simulink model "test"  (R2023b)
settings: Solver=VariableStepAuto  StartTime=0.0  StopTime=10.0  RelTol=1e-3
libraries: mcbcontrolslib x3, dspfdesign x3, slpidlib x3, spsSawtoothGeneratorLib x1, simulink x1, spsSVPWMGenerator2LevelLib x1
settings Model: Creator=LZQ  LastModifiedBy=LZQ

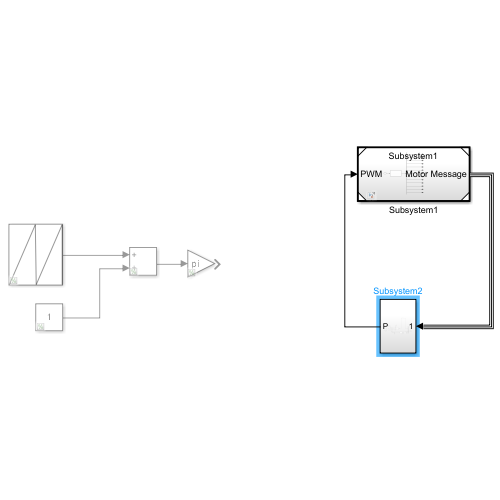
[thumbnail: Simulink's stored preview of the top-level diagram]
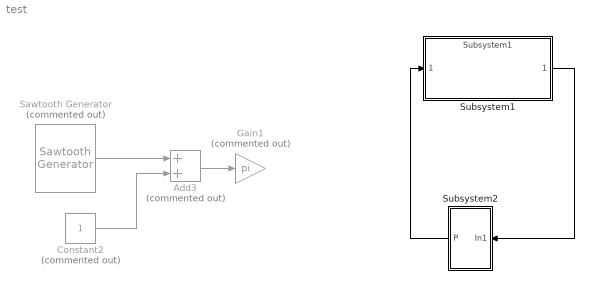
== system test ==
  Add3 : Sum  Commented=on
  Constant2 : Constant  Commented=on
  Gain1 : Gain  Commented=on  Gain=pi
  Sawtooth Generator : spsSawtoothGeneratorLib/Sawtooth Generator  Commented=on  Freq=1  Phase=360  Ts=0
  Subsystem1 : ModelReference  ModelNameDialog=Subsystem1  SimulationMode=Normal  ModelReferenceVersion=1.2
  Subsystem2 : Subsystem
  wires:
  Constant2/1 -> Add3/2
  Add3/1 -> Gain1/1
  Sawtooth Generator/1 -> Add3/1
  Subsystem1/1 -> Subsystem2/1(In1)
  Subsystem2/1(P) -> Subsystem1/1

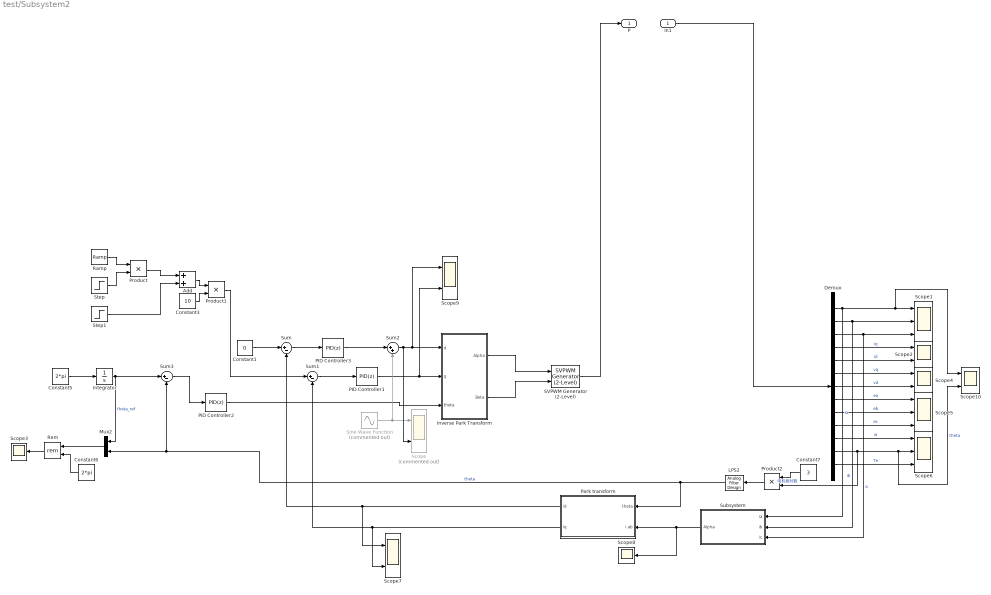
== system test/Subsystem2 ==
  In1 : Inport
  Add : Sum
  Constant1 : Constant  Value=0
  Constant3 : Constant  Value=10
  Constant5 : Constant  Value=2*pi
  Constant6 : Constant  Value=2*pi
  Constant7 : Constant  Value=3
  Demux : Demux  Outputs=13
  Integrator : Integrator
  Inverse Park Transform : Subsystem
  LPS2 : dspfdesign/Analog Filter Design  method=Butterworth  filttype=Lowpass  N=8  Wlo=30  Whi=80  Rp=2  Rs=40
  Mux2 : Mux  Inputs=2
  PID Controller1 : slpidlib/PID Controller  Controller=PID  Form=Parallel  TimeDomain=Discrete-time  UseExternalTs=off  SampleTime=1e-5  IntegratorMethod=Forward Euler  FilterMethod=Forward Euler  ControllerParametersSource=internal  P=0.000004  I=0.000001  UseKiTs=off  D=0  N=100  UseFilter=on  TunerSelectOption=Transfer Function Based (PID Tuner App)  InitialConditionSource=internal  InitialConditionForIntegrator=0  InitialConditionForFilter=0  DifferentiatorICPrevScaledInput=0  ExternalReset=none  TrackingMode=off  Kt=1  LimitOutput=off  SatLimitsSource=internal  UpperSaturationLimit=inf  LowerSaturationLimit=-inf  LinearizeAsGain=on  AntiWindupMode=none  Kb=1  LimitIntegrator=off  UpperIntegratorSaturationLimit=inf  LowerIntegratorSaturationLimit=-inf  POutMin=[]  POutMax=[]  IOutMin=[-0.001]  IOutMax=[0.001]  DOutMin=[]  DOutMax=[]  NOutMin=[]  NOutMax=[]  SumOutMin=[-0.01]  SumOutMax=[0.01]  SaturationOutMin=[]  SaturationOutMax=[]  PParamMin=[]  PParamMax=[]  IParamMin=[]  IParamMax=[]  DParamMin=[]  DParamMax=[]  NParamMin=[]  NParamMax=[]  KbParamMin=[]  KbParamMax=[]  KtParamMin=[]  KtParamMax=[]  KbOutMin=[]  KbOutMax=[]  KtOutMin=[]  KtOutMax=[]  IntegratorOutMin=[]  IntegratorOutMax=[]  FilterOutMin=[]  FilterOutMax=[]  SumI1OutMin=[]  SumI1OutMax=[]  SumI2OutMin=[]  SumI2OutMax=[]  SumI3OutMin=[]  SumI3OutMax=[]  SumI4OutMin=[]  SumI4OutMax=[]  SumDOutMin=[]  SumDOutMax=[]  DifferentiatorOutMin=[]  DifferentiatorOutMax=[]  FilterDiffOutCoefMin=[]  FilterDiffOutCoefMax=[]  ReciprocalOutMin=[]  ReciprocalOutMax=[]  SumDenOutMin=[]  SumDenOutMax=[]  SumNumOutMin=[]  SumNumOutMax=[]  DivideOutMin=[]  DivideOutMax=[]  UdiffTsProdOutMin=[]  UdiffTsProdOutMax=[]  NTsProdOutMin=[]  NTsProdOutMax=[]  UintegralTsProdOutMin=[]  UintegralTsProdOutMax=[]  UngainTsProdOutMin=[]  UngainTsProdOutMax=[]  ClampingZeroOutDataTypeStr=Inherit: Inherit via back propagation  ClampingZeroOutMin=[]  ClampingZeroOutMax=[]  FilterDenConstantOutDataTypeStr=Inherit: Inherit via back propagation  FilterDenConstantOutMin=[]  FilterDenConstantOutMax=[]  PCopyOutDataTypeStr=Inherit: Inherit via back propagation  PCopyOutMin=[]  PCopyOutMax=[]  NCopyOutDataTypeStr=Inherit: Inherit via back propagation  NCopyOutMin=[]  NCopyOutMax=[]  IntegratorContinuousStateAttributes=''  IntegratorStateMustResolveToSignalObject=off  IntegratorRTWStateStorageClass=Auto  FilterContinuousStateAttributes=''  FilterStateMustResolveToSignalObject=off  FilterRTWStateStorageClass=Auto  ParallelPVariant=InternalParameters  IdealPVariant=Disabled  IVariant=InternalParameters  DVariant=InternalParameters  IntegratorVariant=Discrete  SatVariant=Disabled  AWVariant=Passthrough  PCopyVariant=Disabled  TRVariant=Disabled  FdbkBlocksVariant=Forward  IdealPFdbkVariant=Disabled  SatFdbkVariant=Disabled  DerivativeFilterVariant=ForwardEulerFilter  NVariant=InternalParameters  NCopyVariant=Disabled  FilterICVariant=InternalICsFilter  IntegratorICVariant=InternalICs  ExternalResetVariant=Disabled  TRSumVariant=Passthrough  SumFdbkVariant=Disabled  SumVariant=Sum_PID  TsampFilterVariant=InternalTs  TsampNgainVariant=Passthrough  TsampIntegralVariant=Disabled_SignalSpec  ExternalSaturationOutDataTypeStr=Inherit: Same as second input
  PID Controller2 : slpidlib/PID Controller  Controller=PID  Form=Parallel  TimeDomain=Discrete-time  UseExternalTs=off  SampleTime=0.0005  IntegratorMethod=Forward Euler  FilterMethod=Forward Euler  ControllerParametersSource=internal  P=0.1  I=0.04  UseKiTs=off  D=0  N=100  UseFilter=on  TunerSelectOption=Transfer Function Based (PID Tuner App)  InitialConditionSource=internal  InitialConditionForIntegrator=0  InitialConditionForFilter=0  DifferentiatorICPrevScaledInput=0  ExternalReset=none  TrackingMode=off  Kt=1  LimitOutput=off  SatLimitsSource=internal  UpperSaturationLimit=inf  LowerSaturationLimit=-inf  LinearizeAsGain=on  AntiWindupMode=none  Kb=1  LimitIntegrator=off  UpperIntegratorSaturationLimit=inf  LowerIntegratorSaturationLimit=-inf  POutMin=[]  POutMax=[]  IOutMin=[]  IOutMax=[]  DOutMin=[]  DOutMax=[]  NOutMin=[]  NOutMax=[]  SumOutMin=[]  SumOutMax=[]  SaturationOutMin=[]  SaturationOutMax=[]  PParamMin=[]  PParamMax=[]  IParamMin=[]  IParamMax=[]  DParamMin=[]  DParamMax=[]  NParamMin=[]  NParamMax=[]  KbParamMin=[]  KbParamMax=[]  KtParamMin=[]  KtParamMax=[]  KbOutMin=[]  KbOutMax=[]  KtOutMin=[]  KtOutMax=[]  IntegratorOutMin=[]  IntegratorOutMax=[]  FilterOutMin=[]  FilterOutMax=[]  SumI1OutMin=[]  SumI1OutMax=[]  SumI2OutMin=[]  SumI2OutMax=[]  SumI3OutMin=[]  SumI3OutMax=[]  SumI4OutMin=[]  SumI4OutMax=[]  SumDOutMin=[]  SumDOutMax=[]  DifferentiatorOutMin=[]  DifferentiatorOutMax=[]  FilterDiffOutCoefMin=[]  FilterDiffOutCoefMax=[]  ReciprocalOutMin=[]  ReciprocalOutMax=[]  SumDenOutMin=[]  SumDenOutMax=[]  SumNumOutMin=[]  SumNumOutMax=[]  DivideOutMin=[]  DivideOutMax=[]  UdiffTsProdOutMin=[]  UdiffTsProdOutMax=[]  NTsProdOutMin=[]  NTsProdOutMax=[]  UintegralTsProdOutMin=[]  UintegralTsProdOutMax=[]  UngainTsProdOutMin=[]  UngainTsProdOutMax=[]  ClampingZeroOutDataTypeStr=Inherit: Inherit via back propagation  ClampingZeroOutMin=[]  ClampingZeroOutMax=[]  FilterDenConstantOutDataTypeStr=Inherit: Inherit via back propagation  FilterDenConstantOutMin=[]  FilterDenConstantOutMax=[]  PCopyOutDataTypeStr=Inherit: Inherit via back propagation  PCopyOutMin=[]  PCopyOutMax=[]  NCopyOutDataTypeStr=Inherit: Inherit via back propagation  NCopyOutMin=[]  NCopyOutMax=[]  IntegratorContinuousStateAttributes=''  IntegratorStateMustResolveToSignalObject=off  IntegratorRTWStateStorageClass=Auto  FilterContinuousStateAttributes=''  FilterStateMustResolveToSignalObject=off  FilterRTWStateStorageClass=Auto  ParallelPVariant=InternalParameters  IdealPVariant=Disabled  IVariant=InternalParameters  DVariant=InternalParameters  IntegratorVariant=Discrete  SatVariant=Disabled  AWVariant=Passthrough  PCopyVariant=Disabled  TRVariant=Disabled  FdbkBlocksVariant=Forward  IdealPFdbkVariant=Disabled  SatFdbkVariant=Disabled  DerivativeFilterVariant=ForwardEulerFilter  NVariant=InternalParameters  NCopyVariant=Disabled  FilterICVariant=InternalICsFilter  IntegratorICVariant=InternalICs  ExternalResetVariant=Disabled  TRSumVariant=Passthrough  SumFdbkVariant=Disabled  SumVariant=Sum_PID  TsampFilterVariant=InternalTs  TsampNgainVariant=Passthrough  TsampIntegralVariant=Disabled_SignalSpec  ExternalSaturationOutDataTypeStr=Inherit: Same as second input
  PID Controller3 : slpidlib/PID Controller  Controller=PID  Form=Parallel  TimeDomain=Discrete-time  UseExternalTs=off  SampleTime=1e-5  IntegratorMethod=Forward Euler  FilterMethod=Forward Euler  ControllerParametersSource=internal  P=0.000004  I=0.000001  UseKiTs=off  D=0  N=100  UseFilter=on  TunerSelectOption=Transfer Function Based (PID Tuner App)  InitialConditionSource=internal  InitialConditionForIntegrator=0  InitialConditionForFilter=0  DifferentiatorICPrevScaledInput=0  ExternalReset=none  TrackingMode=off  Kt=1  LimitOutput=off  SatLimitsSource=internal  UpperSaturationLimit=inf  LowerSaturationLimit=-inf  LinearizeAsGain=on  AntiWindupMode=none  Kb=1  LimitIntegrator=off  UpperIntegratorSaturationLimit=inf  LowerIntegratorSaturationLimit=-inf  POutMin=[]  POutMax=[]  IOutMin=[-0.001]  IOutMax=[0.001]  DOutMin=[]  DOutMax=[]  NOutMin=[]  NOutMax=[]  SumOutMin=[-0.01]  SumOutMax=[0.01]  SaturationOutMin=[]  SaturationOutMax=[]  PParamMin=[]  PParamMax=[]  IParamMin=[]  IParamMax=[]  DParamMin=[]  DParamMax=[]  NParamMin=[]  NParamMax=[]  KbParamMin=[]  KbParamMax=[]  KtParamMin=[]  KtParamMax=[]  KbOutMin=[]  KbOutMax=[]  KtOutMin=[]  KtOutMax=[]  IntegratorOutMin=[]  IntegratorOutMax=[]  FilterOutMin=[]  FilterOutMax=[]  SumI1OutMin=[]  SumI1OutMax=[]  SumI2OutMin=[]  SumI2OutMax=[]  SumI3OutMin=[]  SumI3OutMax=[]  SumI4OutMin=[]  SumI4OutMax=[]  SumDOutMin=[]  SumDOutMax=[]  DifferentiatorOutMin=[]  DifferentiatorOutMax=[]  FilterDiffOutCoefMin=[]  FilterDiffOutCoefMax=[]  ReciprocalOutMin=[]  ReciprocalOutMax=[]  SumDenOutMin=[]  SumDenOutMax=[]  SumNumOutMin=[]  SumNumOutMax=[]  DivideOutMin=[]  DivideOutMax=[]  UdiffTsProdOutMin=[]  UdiffTsProdOutMax=[]  NTsProdOutMin=[]  NTsProdOutMax=[]  UintegralTsProdOutMin=[]  UintegralTsProdOutMax=[]  UngainTsProdOutMin=[]  UngainTsProdOutMax=[]  ClampingZeroOutDataTypeStr=Inherit: Inherit via back propagation  ClampingZeroOutMin=[]  ClampingZeroOutMax=[]  FilterDenConstantOutDataTypeStr=Inherit: Inherit via back propagation  FilterDenConstantOutMin=[]  FilterDenConstantOutMax=[]  PCopyOutDataTypeStr=Inherit: Inherit via back propagation  PCopyOutMin=[]  PCopyOutMax=[]  NCopyOutDataTypeStr=Inherit: Inherit via back propagation  NCopyOutMin=[]  NCopyOutMax=[]  IntegratorContinuousStateAttributes=''  IntegratorStateMustResolveToSignalObject=off  IntegratorRTWStateStorageClass=Auto  FilterContinuousStateAttributes=''  FilterStateMustResolveToSignalObject=off  FilterRTWStateStorageClass=Auto  ParallelPVariant=InternalParameters  IdealPVariant=Disabled  IVariant=InternalParameters  DVariant=InternalParameters  IntegratorVariant=Discrete  SatVariant=Disabled  AWVariant=Passthrough  PCopyVariant=Disabled  TRVariant=Disabled  FdbkBlocksVariant=Forward  IdealPFdbkVariant=Disabled  SatFdbkVariant=Disabled  DerivativeFilterVariant=ForwardEulerFilter  NVariant=InternalParameters  NCopyVariant=Disabled  FilterICVariant=InternalICsFilter  IntegratorICVariant=InternalICs  ExternalResetVariant=Disabled  TRSumVariant=Passthrough  SumFdbkVariant=Disabled  SumVariant=Sum_PID  TsampFilterVariant=InternalTs  TsampNgainVariant=Passthrough  TsampIntegralVariant=Disabled_SignalSpec  ExternalSaturationOutDataTypeStr=Inherit: Same as second input
  Park transform : Subsystem
  Product : Product
  Product1 : Product
  Product2 : Product
  Ramp : simulink/Sources/Ramp  slope=0.2  start=0  InitialOutput=0.2
  Rem : Math  Operator=rem
  SVPWM Generator (2-Level) : spsSVPWMGenerator2LevelLib/SVPWM Generator (2-Level)  InputType=alpha-beta components  SwitchingPattern=Pattern #1  Fc=20000  ParUref=[0.8 -30 50]  Ts=0
  Scope : Scope  Commented=on  NumInputPorts=2
  Scope1 : Scope  NumInputPorts=3
  Scope{2,4,7,9..10} (5 alike) : Scope  NumInputPorts=2
  Scope3 : Scope
  Scope5 : Scope  NumInputPorts=3
  Scope6 : Scope  NumInputPorts=3
  Scope8 : Scope
  Sine Wave Function : Sin  Commented=on  Amplitude=0.2  Frequency=2*pi*800  Phase=pi/2  SampleTime=0.000005
  Step : Step  Time=4  Before=1  After=0  SampleTime=0
  Step1 : Step  Time=4  SampleTime=0
  Subsystem : Subsystem
  Sum : Sum  Inputs=|+-
  Sum1 : Sum  Inputs=|+-
  Sum2 : Sum  Inputs=|++
  Sum3 : Sum  Inputs=|+-
  P : Outport
  wires:
  PID Controller2/1 -> Inverse Park Transform/3(theta)
  Demux/1 -> Subsystem/1(ia), Scope10/1, Scope1/1  "ia"
  PID Controller1/1 -> Scope9/2, Inverse Park Transform/2(q)
  LPS2/1 -> Sum3/2, Mux2/2, Park transform/1(theta)  "theta"
  Inverse Park Transform/1(Alpha) -> SVPWM Generator (2-Level)/1
  Sine Wave Function/1 -> Sum2/2, Scope/1
  Demux/9 -> Scope5/2  "eb"
  Rem/1 -> Scope3/1
  Constant3/1 -> Product1/2
  Sum2/1 -> Scope9/1, Inverse Park Transform/1(d), Scope/2
  Demux/7 -> Scope4/2  "vd"
  Inverse Park Transform/2(Beta) -> SVPWM Generator (2-Level)/2
  Constant1/1 -> Sum/1
  Product/1 -> Add/1
  PID Controller3/1 -> Sum2/1
  Park transform/2(iq) -> Sum1/2, Scope7/2
  Sum1/1 -> PID Controller1/1
  Sum3/1 -> PID Controller2/1
  Constant7/1 -> Product2/1  "电机极对数"
  Park transform/1(id) -> Sum/2, Scope7/1
  Demux/12 -> Product2/2, Scope10/2, Scope6/2  "theta"
  Constant5/1 -> Integrator/1
  Add/1 -> Product1/1
  Demux/3 -> Subsystem/3(ic), Scope1/3  "ic"
  Integrator/1 -> Mux2/1, Sum3/1  "theta_ref"
  Demux/4 -> Scope2/1  "iq"
  Demux/2 -> Subsystem/2(ib), Scope1/2  "ib"
  Step1/1 -> Add/2
  Demux/13 -> Scope6/3  "Te"
  Subsystem/1(Alpha) -> Park transform/2(i ab), Scope8/1
  Ramp/1 -> Product/1
  Demux/10 -> Scope5/3  "ec"
  Mux2/1 -> Rem/1
  Constant6/1 -> Rem/2
  Demux/11 -> Scope6/1  "w"
  Demux/6 -> Scope4/1  "vq"
  Demux/5 -> Scope2/2  "id"
  Demux/8 -> Scope5/1  "ea"
  Product1/1 -> Sum1/1
  Sum/1 -> PID Controller3/1
  Step/1 -> Product/2
  Product2/1 -> LPS2/1
  SVPWM Generator (2-Level)/1 -> P/1
  In1/1 -> Demux/1

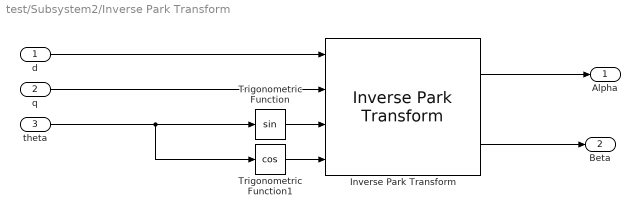
== system test/Subsystem2/Inverse Park Transform ==
  d : Inport  SampleTime=1e-5
  q : Inport  Port=2  SampleTime=1e-5
  theta : Inport  Port=3
  Inverse Park Transform : mcbcontrolslib/Inverse Park Transform  PhaseInput=Two inputs  AxisAlignment=D-axis  ThetaInput=Sine and Cosine electrical position  AngleInput=Per-unit  N_points=1024
      settings: LibrarySourceBlock=mcblib/Controls/Math Transforms/Inverse Park Transform
  Trigonometric Function : Trigonometry
  Trigonometric Function1 : Trigonometry  Operator=cos
  Alpha : Outport
  Beta : Outport  Port=2
  wires:
  theta/1 -> Trigonometric Function1/1, Trigonometric Function/1
  Trigonometric Function1/1 -> Inverse Park Transform/4
  Trigonometric Function/1 -> Inverse Park Transform/3
  Inverse Park Transform/1 -> Alpha/1
  d/1 -> Inverse Park Transform/1
  q/1 -> Inverse Park Transform/2
  Inverse Park Transform/2 -> Beta/1

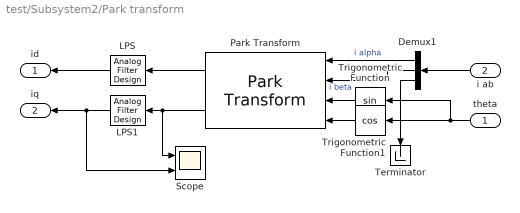
== system test/Subsystem2/Park transform ==
  theta : Inport  SampleTime=1e-5
  i ab : Inport  Port=2  SampleTime=1e-5
  Demux1 : Demux  Outputs=3
  LPS : dspfdesign/Analog Filter Design  method=Butterworth  filttype=Lowpass  N=3  Wlo=500  Whi=80  Rp=2  Rs=40
  LPS1 : dspfdesign/Analog Filter Design  method=Butterworth  filttype=Lowpass  N=3  Wlo=500  Whi=80  Rp=2  Rs=40
  Park Transform : mcbcontrolslib/Park Transform  PhaseInput=Two inputs  AxisAlignment=D-axis  ThetaInput=Sine and Cosine electrical position  AngleInput=Per-unit  N_points=1024
      settings: LibrarySourceBlock=mcblib/Controls/Math Transforms/Park Transform
  Scope : Scope  NumInputPorts=2
  Terminator : Terminator
  Trigonometric Function : Trigonometry
  Trigonometric Function1 : Trigonometry  Operator=cos
  id : Outport  SampleTime=1e-5
  iq : Outport  Port=2  SampleTime=1e-5
  wires:
  Demux1/3 -> Terminator/1
  Trigonometric Function1/1 -> Park Transform/4
  theta/1 -> Trigonometric Function/1, Trigonometric Function1/1
  Park Transform/1 -> LPS/1
  LPS/1 -> id/1
  Park Transform/2 -> Scope/1, LPS1/1
  Demux1/2 -> Park Transform/2  "i beta"
  Demux1/1 -> Park Transform/1  "i alpha"
  Trigonometric Function/1 -> Park Transform/3
  i ab/1 -> Demux1/1
  LPS1/1 -> iq/1, Scope/2

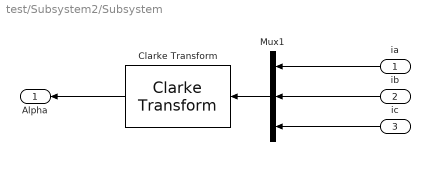
== system test/Subsystem2/Subsystem ==
  ia : Inport  SampleTime=1e-5
  ib : Inport  Port=2  SampleTime=1e-5
  ic : Inport  Port=3  SampleTime=1e-5
  Clarke Transform : mcbcontrolslib/Clarke Transform  VariantControl=Variant2  PhaseInput=Three inputs  EnPowerInv=off
      settings: LibrarySourceBlock=mcblib/Controls/Math Transforms/Clarke Transform
  Mux1 : Mux  Inputs=3
  Alpha : Outport  SampleTime=1e-5
  wires:
  Mux1/1 -> Clarke Transform/1
  ia/1 -> Mux1/1
  ib/1 -> Mux1/2
  Clarke Transform/1 -> Alpha/1
  ic/1 -> Mux1/3
